simulink model "Problem1_8"  (R2018a)
settings: Solver=VariableStepAuto  StartTime=0.0  StopTime=30  RelTol=1e-3
settings Model: Creator=NIMA  LastModifiedBy=NIMA

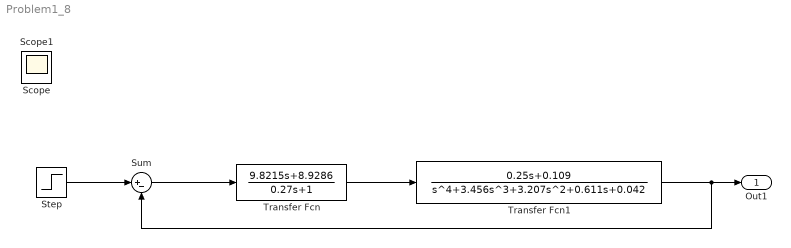
== system Problem1_8 ==
  Step : Step  SampleTime=0
  Sum : Sum  Inputs=|+-
  Transfer Fcn : TransferFcn  Numerator=[9.8215 8.9286]  Denominator=[0.27 1]
  Transfer Fcn1 : TransferFcn  Numerator=[0.25 0.109]  Denominator=[1 3.456 3.207 0.611 0.042]
  Out1 : Outport
  Scope : Scope
  Scope1 : Scope
  wires:
  Transfer Fcn/1 -> Transfer Fcn1/1
  Transfer Fcn1/1 -> Sum/2, Out1/1
  Sum/1 -> Transfer Fcn/1
  Step/1 -> Sum/1
